simulink model "tvg_bee_v03"  (Simulink 6.2)
settings: Solver=ode45  StartTime=0.0  StopTime=60  RelTol=1e-3
libraries: xbsIndex_r3 x53, xps_library x7, casper_library x2
settings Model: LastModifiedBy=lspitler
settings DebuggingCC: SolverPrmCheckMsg=warning

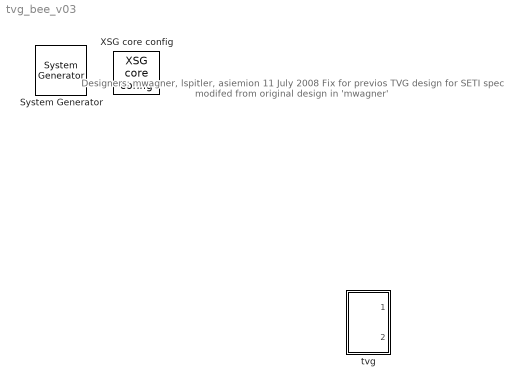
== system tvg_bee_v03 ==
  note: Designers: mwagner, lspitler, asiemion
      | 11 July 2008
      | Fix for previos TVG design for SETI spec
      | modifed from original design in 'mwagner'
  " System Generator" : xbsIndex_r3/ System Generator  Tag=genX  xilinxfamily=Virtex2P  part=xc2vp70  speed=-7  package=ff1704  synthesis_tool=XST  directory=./tvg_bee_v03/sysgen  testbench=off  simulink_period=1  sysclk_period=10  incr_netlist=off  trim_vbits=Everywhere in SubSystem  dbl_ovrd=According to Block Masks  core_generation=According to Block Masks  run_coregen=off  deprecated_control=off  eval_field=0
      settings: AttributesFormatString=System\nGenerator
  XSG core config : xps_library/XSG core config  Tag=xps:xsg  hw_sys=BEE2_usr  ibob_linux=off  clk_src=sys_clk  gpio_clk_io_group=iBOB:sma  gpio_clk_bit_index=0  clk_rate=100  sample_period=1  synthesis_tool=XST  mpc_type=powerpc405
  tvg : Subsystem

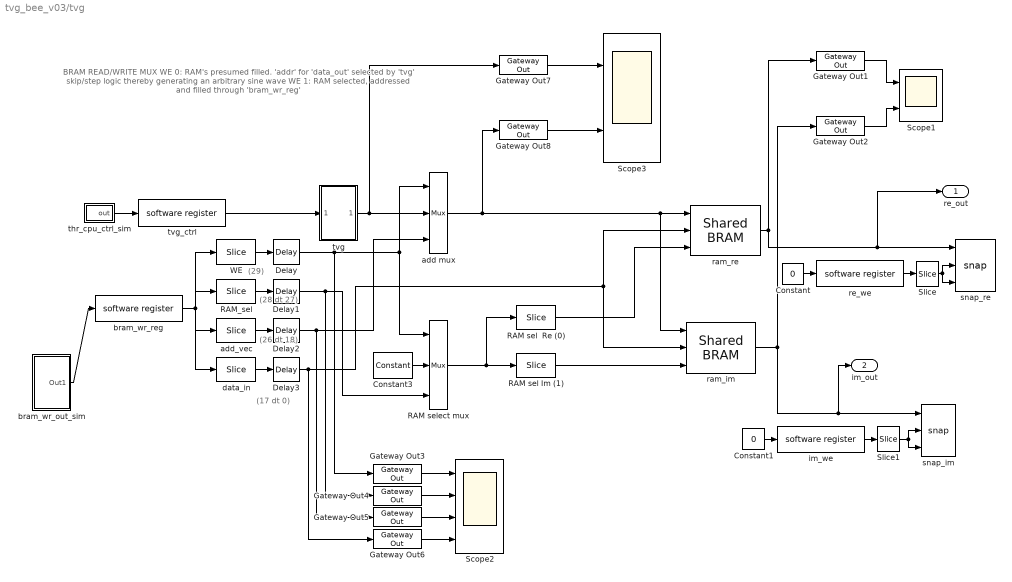
== system tvg_bee_v03/tvg ==
  note: BRAM READ/WRITE MUX
      | WE 0: RAM's presumed filled.
      | 'addr' for 'data_out' selected
      | by 'tvg' skip/step logic thereby
      | generating an arbitrary sine wave
      | WE 1: RAM selected, addressed
      | and filled through
      | 'bram_wr_reg'
  note: (29)
  note: (28 dt 27)
  note: (17 dt 0)
  note: (26 dt 18)
  Constant : Constant  Value=0
  Constant1 : Constant  Value=0
  Constant3 : xbsIndex_r3/Constant  const=0  equ=P=C  arith_type=Unsigned  n_bits=4  bin_pt=0  opselect=C  inp2=PCIN>>17  opr=+  inp1=P  carry=CIN  iostate=0  explicit_period=on  period=1  dbl_ovrd=off
  Delay{,1..3} (4 alike) : xbsIndex_r3/Delay  latency=1  reg_retiming=off  explicit_period=on  period=1  en=off  accept_only_valid=off  init_zero=on  dbl_ovrd=off  show_param=off
      settings: xl_area=[0, 0, 0, 0, 0, 0, 0]
  Gateway Out{1..8} (8 alike) : xbsIndex_r3/Gateway Out  output_type=Double  nbits=8  bin_pt=6  arith_type=Boolean  quantization=Truncate  overflow=Wrap  hdl_port=on  timing_constraint=None  locs_specified=off  LOCs={}  needs_fixed_name=off  show_param=off
      settings: xl_area=[0, 0, 0, 0, 0, 0, 0]
  RAM sel  Re (0) : xbsIndex_r3/Slice  mode=Lower Bit Location + Width  nbits=1  bit1=0  base1=MSB of Input  bit0=0  base0=LSB of Input  boolean_output=on  explicit_period=on  period=1  dbl_ovrd=off
  RAM sel Im (1) : xbsIndex_r3/Slice  mode=Lower Bit Location + Width  nbits=1  bit1=0  base1=MSB of Input  bit0=1  base0=LSB of Input  boolean_output=on  explicit_period=on  period=1  dbl_ovrd=off
  RAM select mux : xbsIndex_r3/Mux  inputs=2  precision=Full  arith_type="Signed  (2's comp)"  n_bits=8  bin_pt=2  quantization=Truncate  overflow=Wrap  latency=0  explicit_period=on  period=1  en=off  dbl_ovrd=off  show_param=off  mux_type=off  use_rpm=off  gen_core=off
      settings: xl_area=[0, 0, 0, 0, 0, 0, 0]
  RAM_sel : xbsIndex_r3/Slice  mode=Lower Bit Location + Width  nbits=2  bit1=10  base1=MSB of Input  bit0=27  base0=LSB of Input  boolean_output=off  explicit_period=on  period=1  dbl_ovrd=off
  Scope1 : Scope  NumInputPorts=2
      settings: YMin=-5~-5  YMax=5~5  SaveName=ScopeData2
  Scope2 : Scope  NumInputPorts=4
      settings: YMin=-5~-5~-5~-5  YMax=5~5~5~5
  Scope3 : Scope  NumInputPorts=2
      settings: YMin=-5~-5  YMax=5~5  SaveName=ScopeData3
  Slice : xbsIndex_r3/Slice  mode=Lower Bit Location + Width  nbits=1  bit1=0  base1=MSB of Input  bit0=0  base0=LSB of Input  boolean_output=on  explicit_period=off  period=1  dbl_ovrd=off
  Slice1 : xbsIndex_r3/Slice  mode=Lower Bit Location + Width  nbits=1  bit1=0  base1=MSB of Input  bit0=0  base0=LSB of Input  boolean_output=on  explicit_period=off  period=1  dbl_ovrd=off
  WE : xbsIndex_r3/Slice  mode=Lower Bit Location + Width  nbits=1  bit1=10  base1=MSB of Input  bit0=29  base0=LSB of Input  boolean_output=off  explicit_period=on  period=1  dbl_ovrd=off
  add mux : xbsIndex_r3/Mux  inputs=2  precision=Full  arith_type="Signed  (2's comp)"  n_bits=8  bin_pt=2  quantization=Truncate  overflow=Wrap  latency=0  explicit_period=on  period=1  en=off  dbl_ovrd=off  show_param=off  mux_type=off  use_rpm=off  gen_core=off
      settings: xl_area=[0, 0, 0, 0, 0, 0, 0]
  add_vec : xbsIndex_r3/Slice  mode=Lower Bit Location + Width  nbits=9  bit1=0  base1=MSB of Input  bit0=18  base0=LSB of Input  boolean_output=off  explicit_period=on  period=1  dbl_ovrd=off
  bram_wr_out_sim : Subsystem  mask{we_enable=0, ram_sel=3, add_vec=512, data_in=32}
      mask prompts: we_enable "Write enable"; ram_sel "RAM selector (1 = Re; 2 = Im; 3 = both)"; add_vec "RAM address"; data_in "Data in"
  bram_wr_reg : xps_library/software register  Tag=xps:sw_reg  io_dir=From Processor  arith_type=Unsigned  bitwidth=32  bin_pt=0  sample_period=1  gw_name=tvg_bee_v03_bram_wr_reg_user_data_out
  data_in : xbsIndex_r3/Slice  mode=Lower Bit Location + Width  nbits=18  bit1=0  base1=MSB of Input  bit0=0  base0=LSB of Input  boolean_output=off  explicit_period=on  period=1  dbl_ovrd=off
  im_we : xps_library/software register  Tag=xps:sw_reg  io_dir=From Processor  arith_type=Unsigned  bitwidth=32  bin_pt=0  sample_period=1  gw_name=tvg_bee_v03_im_we_user_data_out
  ram_im : xps_library/Shared BRAM  Tag=xps:bram  arith_type="Signed  (2's comp)"  addr_width=11  data_width=32  data_bin_pt=0  init_vals=[1:2^11]  sample_rate=1
  ram_re : xps_library/Shared BRAM  Tag=xps:bram  arith_type="Signed  (2's comp)"  addr_width=11  data_width=32  data_bin_pt=0  init_vals=[1:2^11]  sample_rate=1
  re_we : xps_library/software register  Tag=xps:sw_reg  io_dir=From Processor  arith_type=Unsigned  bitwidth=32  bin_pt=0  sample_period=1  gw_name=tvg_bee_v03_re_we_user_data_out
  snap_im : casper_library/Scopes/snap  nsamples=11
  snap_re : casper_library/Scopes/snap  nsamples=11
  thr_cpu_ctrl_sim : Subsystem  mask{tvg_skip=1, tvg_stall=2, tvg_length=5}
      mask prompts: tvg_skip "Skip"; tvg_stall "Stall"; tvg_length "Length"
      mask help:
      | Mux Data for CT and FFT Syncs:
      |
      | 0 -> Interchip Connection
      | 1 -> User Generated External Sync
      | 2 -> Periodic Sync Generator
      | 3 -> Periodic Sync Generator (Same as 2)
      |
      | Mux Data for CT and FFT Inputs:
      |
      | 0 -> Interchip Connection
      | 1 -> Test Vector Generator (TVG)
      | 2 -> All Zeroes (0's)
      | 3 -> All Ones (1's)
  tvg : Subsystem  mask(Test Vector Generator(TVG)){tvg_skip=1, tvg_stall=1, tvg_length=512}
      mask prompts: tvg_skip "Skip"; tvg_stall "Stall"; tvg_length "Length"
  tvg_ctrl : xps_library/software register  Tag=xps:sw_reg  io_dir=From Processor  arith_type=Unsigned  bitwidth=32  bin_pt=0  sample_period=1  gw_name=tvg_bee_v03_tvg_ctrl_user_data_out
  re_out : Outport
  im_out : Outport  Port=2
  wires:
  tvg_ctrl/1 -> tvg/1(In1)
  tvg/1(Out1) -> add mux/2, Gateway Out7/1
  Constant3/1 -> RAM select mux/2
  RAM select mux/1 -> RAM sel  Re (0)/1, RAM sel Im (1)/1
  RAM sel  Re (0)/1 -> ram_re/3
  WE/1 -> Delay/1
  Gateway Out1/1 -> Scope1/1
  Gateway Out2/1 -> Scope1/2
  thr_cpu_ctrl_sim/1(out) -> tvg_ctrl/1
  bram_wr_reg/1 -> data_in/1, add_vec/1, RAM_sel/1, WE/1
  add_vec/1 -> Delay2/1
  RAM_sel/1 -> Delay1/1
  add mux/1 -> ram_im/1, ram_re/1, Gateway Out8/1
  data_in/1 -> Delay3/1
  RAM sel Im (1)/1 -> ram_im/3
  ram_re/1 -> Gateway Out1/1, snap_re/1, re_out/1
  ram_im/1 -> Gateway Out2/1, snap_im/1, im_out/1
  bram_wr_out_sim/1(Out1) -> bram_wr_reg/1
  Gateway Out3/1 -> Scope2/1
  Gateway Out4/1 -> Scope2/2
  Gateway Out5/1 -> Scope2/3
  Gateway Out6/1 -> Scope2/4
  Delay/1 -> Gateway Out3/1, add mux/1, RAM select mux/1
  Delay1/1 -> Gateway Out4/1, RAM select mux/3
  Delay2/1 -> Gateway Out5/1, add mux/3
  Delay3/1 -> Gateway Out6/1, ram_re/2, ram_im/2
  Gateway Out7/1 -> Scope3/1
  Gateway Out8/1 -> Scope3/2
  Slice/1 -> snap_re/2, snap_re/3
  re_we/1 -> Slice/1
  Constant/1 -> re_we/1
  Slice1/1 -> snap_im/2, snap_im/3
  im_we/1 -> Slice1/1
  Constant1/1 -> im_we/1

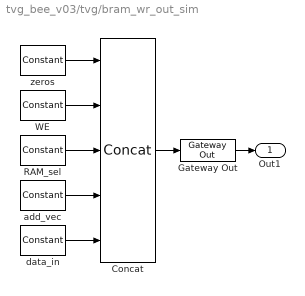
== system tvg_bee_v03/tvg/bram_wr_out_sim ==
  Concat : xbsIndex_r3/Concat  num_inputs=5  explicit_period=off  period=1  dbl_ovrd=off
  Gateway Out : xbsIndex_r3/Gateway Out  output_type=Double  nbits=8  bin_pt=6  arith_type=Boolean  quantization=Truncate  overflow=Wrap  hdl_port=on  timing_constraint=None  locs_specified=off  LOCs={}  needs_fixed_name=off  show_param=off
      settings: xl_area=[0, 0, 0, 0, 0, 0, 0]
  RAM_sel : xbsIndex_r3/Constant  const=ram_sel  equ=P=C  arith_type=Unsigned  n_bits=2  bin_pt=0  opselect=C  inp2=PCIN>>17  opr=+  inp1=P  carry=CIN  iostate=0  explicit_period=on  period=1  dbl_ovrd=off
  WE : xbsIndex_r3/Constant  const=we_enable  equ=P=C  arith_type=Unsigned  n_bits=1  bin_pt=0  opselect=C  inp2=PCIN>>17  opr=+  inp1=P  carry=CIN  iostate=0  explicit_period=on  period=1  dbl_ovrd=off
  add_vec : xbsIndex_r3/Constant  const=add_vec  equ=P=C  arith_type=Unsigned  n_bits=9  bin_pt=0  opselect=C  inp2=PCIN>>17  opr=+  inp1=P  carry=CIN  iostate=0  explicit_period=on  period=1  dbl_ovrd=off
  data_in : xbsIndex_r3/Constant  const=data_in  equ=P=C  arith_type=Unsigned  n_bits=18  bin_pt=0  opselect=C  inp2=PCIN>>17  opr=+  inp1=P  carry=CIN  iostate=0  explicit_period=on  period=1  dbl_ovrd=off
  zeros : xbsIndex_r3/Constant  const=0  equ=P=C  arith_type=Unsigned  n_bits=2  bin_pt=0  opselect=C  inp2=PCIN>>17  opr=+  inp1=P  carry=CIN  iostate=0  explicit_period=on  period=1  dbl_ovrd=off
  Out1 : Outport
  wires:
  Gateway Out/1 -> Out1/1
  Concat/1 -> Gateway Out/1
  zeros/1 -> Concat/1
  WE/1 -> Concat/2
  RAM_sel/1 -> Concat/3
  add_vec/1 -> Concat/4
  data_in/1 -> Concat/5

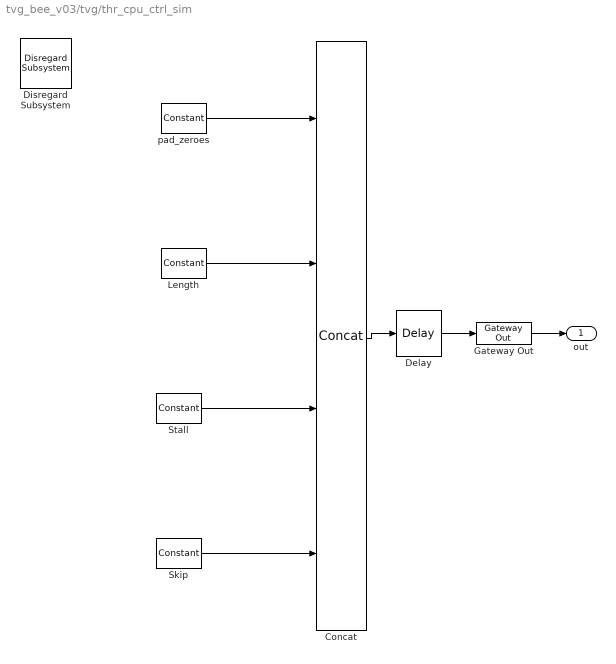
== system tvg_bee_v03/tvg/thr_cpu_ctrl_sim ==
  Concat : xbsIndex_r3/Concat  num_inputs=4  explicit_period=off  period=1  dbl_ovrd=off
  Delay : xbsIndex_r3/Delay  latency=1  reg_retiming=off  explicit_period=off  period=1  en=off  accept_only_valid=off  init_zero=on  dbl_ovrd=off  show_param=off
      settings: xl_area=[0, 0, 0, 0, 0, 0, 0]
  Disregard Subsystem : xbsIndex_r3/Disregard Subsystem  Tag=discardX
      settings: AttributesFormatString=Disregard Subsystem\nFor Generation
  Gateway Out : xbsIndex_r3/Gateway Out  output_type=Double  nbits=8  bin_pt=6  arith_type=Boolean  quantization=Truncate  overflow=Wrap  hdl_port=off  timing_constraint=None  locs_specified=off  LOCs={}  needs_fixed_name=off  show_param=off
      settings: xl_area=[0, 0, 0, 0, 0, 0, 0]
  Length : xbsIndex_r3/Constant  const=tvg_length  equ=P=C  arith_type=Unsigned  n_bits=10  bin_pt=0  opselect=C  inp2=PCIN>>17  opr=+  inp1=P  carry=CIN  iostate=0  explicit_period=on  period=1  dbl_ovrd=off
  "Skip\t" : xbsIndex_r3/Constant  const=tvg_skip  equ=P=C  arith_type=Unsigned  n_bits=10  bin_pt=0  opselect=C  inp2=PCIN>>17  opr=+  inp1=P  carry=CIN  iostate=0  explicit_period=on  period=1  dbl_ovrd=off
  Stall : xbsIndex_r3/Constant  const=tvg_stall  equ=P=C  arith_type=Unsigned  n_bits=10  bin_pt=0  opselect=C  inp2=PCIN>>17  opr=+  inp1=P  carry=CIN  iostate=0  explicit_period=on  period=1  dbl_ovrd=off
  pad_zeroes : xbsIndex_r3/Constant  const=0  equ=P=C  arith_type=Unsigned  n_bits=2  bin_pt=0  opselect=C  inp2=PCIN>>17  opr=+  inp1=P  carry=CIN  iostate=0  explicit_period=on  period=1  dbl_ovrd=off
  out : Outport
  wires:
  "Skip\t"/1 -> Concat/4
  Delay/1 -> Gateway Out/1
  Concat/1 -> Delay/1
  Gateway Out/1 -> out/1
  Stall/1 -> Concat/3
  pad_zeroes/1 -> Concat/1
  Length/1 -> Concat/2

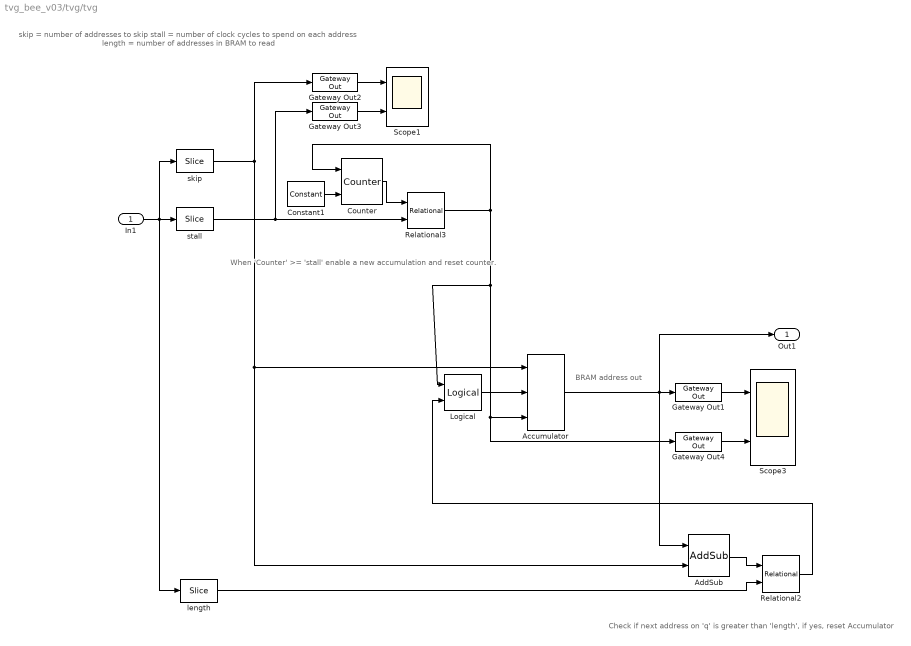
== system tvg_bee_v03/tvg/tvg ==
  note: skip = number of addresses to skip
      | stall = number of clock cycles to spend
      | on each address
      | length = number of addresses in BRAM
      | to read
  note: When 'Counter' >= 'stall'
      | enable a new accumulation
      | and reset counter.
  note: Check if next address on 'q'
      | is greater than 'length',
      | if yes, reset Accumulator
  note: BRAM address out
  In1 : Inport  Port=1  LatchInput=off
  Accumulator : xbsIndex_r3/Accumulator  n_bits=10  overflow=Wrap  operation=Add  scale=1  explicit_period=on  period=1  rst=on  hasbypass=off  en=on  dbl_ovrd=off  show_param=off  gen_core=off  use_rpm=on
      settings: xl_area=[0, 0, 0, 0, 0, 0, 0]
  AddSub : xbsIndex_r3/AddSub  mode=Addition  precision=Full  arith_type=Unsigned  n_bits=8  bin_pt=2  quantization=Truncate  overflow=Wrap  latency=0  explicit_period=on  period=1  use_carryin=off  use_carryout=off  en=off  dbl_ovrd=off  show_param=off  use_core=on  pipeline=off  use_rpm=on  gen_core=off
      settings: xl_area=[0, 0, 0, 0, 0, 0, 0]
  Constant1 : xbsIndex_r3/Constant  const=1  equ=P=C  arith_type=Unsigned  n_bits=10  bin_pt=0  opselect=C  inp2=PCIN>>17  opr=+  inp1=P  carry=CIN  iostate=0  explicit_period=on  period=1  dbl_ovrd=off
  Counter : xbsIndex_r3/Counter  cnt_type=Free Running  n_bits=10  bin_pt=0  arith_type=Unsigned  start_count=0  cnt_to=inf  cnt_by_val=1  operation=Up  explicit_period=on  period=1  load_pin=on  rst=off  en=off  dbl_ovrd=off  show_param=off  use_rpm=on  gen_core=off
      settings: xl_area=[0, 0, 0, 0, 0, 0, 0]
  Gateway Out{1..4} (4 alike) : xbsIndex_r3/Gateway Out  output_type=Double  nbits=8  bin_pt=6  arith_type=Boolean  quantization=Truncate  overflow=Wrap  hdl_port=on  timing_constraint=None  locs_specified=off  LOCs={}  needs_fixed_name=off  show_param=off
      settings: xl_area=[0, 0, 0, 0, 0, 0, 0]
  Logical : xbsIndex_r3/Logical  logical_function=AND  inputs=2  precision=Full  arith_type=Unsigned  n_bits=8  bin_pt=2  align_bp=on  latency=0  explicit_period=off  period=1  en=off  dbl_ovrd=off  show_param=off
      settings: xl_area=[0, 0, 0, 0, 0, 0, 0]
  Relational2 : xbsIndex_r3/Relational  mode=a>=b  latency=0  explicit_period=on  period=1  en=off  dbl_ovrd=off  show_param=off
      settings: xl_area=[0, 0, 0, 0, 0, 0, 0]
  Relational3 : xbsIndex_r3/Relational  mode=a>=b  latency=0  explicit_period=on  period=1  en=off  dbl_ovrd=off  show_param=off
      settings: xl_area=[0, 0, 0, 0, 0, 0, 0]
  Scope1 : Scope  NumInputPorts=2
      settings: YMin=-5~-5  YMax=5~5
  Scope3 : Scope  NumInputPorts=2
      settings: TimeRange=20  YMin=-5~-5  YMax=5~5  SaveName=ScopeData4
  length : xbsIndex_r3/Slice  mode=Lower Bit Location + Width  nbits=10  bit1=0  base1=MSB of Input  bit0=20  base0=LSB of Input  boolean_output=off  explicit_period=on  period=1  dbl_ovrd=off
  skip : xbsIndex_r3/Slice  mode=Lower Bit Location + Width  nbits=10  bit1=0  base1=MSB of Input  bit0=0  base0=LSB of Input  boolean_output=off  explicit_period=on  period=1  dbl_ovrd=off
  stall : xbsIndex_r3/Slice  mode=Lower Bit Location + Width  nbits=10  bit1=0  base1=MSB of Input  bit0=10  base0=LSB of Input  boolean_output=off  explicit_period=on  period=1  dbl_ovrd=off
  Out1 : Outport
  wires:
  length/1 -> Relational2/2
  AddSub/1 -> Relational2/1
  Logical/1 -> Accumulator/2
  Relational2/1 -> Logical/2
  Constant1/1 -> Counter/2
  Counter/1 -> Relational3/1
  Relational3/1 -> Logical/1, Gateway Out4/1, Accumulator/3, Counter/1
  Gateway Out4/1 -> Scope3/2
  Gateway Out3/1 -> Scope1/2
  Gateway Out2/1 -> Scope1/1
  stall/1 -> Relational3/2, Gateway Out3/1
  skip/1 -> AddSub/2, Accumulator/1, Gateway Out2/1
  Accumulator/1 -> Gateway Out1/1, AddSub/1, Out1/1
  Gateway Out1/1 -> Scope3/1
  In1/1 -> length/1, skip/1, stall/1
